simulink model "Adder"  (R2025a)
settings: Solver=FixedStepAuto  StartTime=0.0  StopTime=10.0  RelTol=1e-3
undefined symbols (not defined in the file or in its folder): A, B
libraries: hdlsllib x8
settings Model: Creator=Soochan Kim  LastModifiedBy=Soochan Kim
settings SolverCC: PositivePriorityOrder=on
settings OptimizationCC: BlockReduction=off  ConditionallyExecuteInputs=off  DefaultParameterBehavior=Inlined  EnhancedBackFolding=on  PassReuseOutputArgsAs=Individual arguments  ZeroExternalMemoryAtStartup=off  ZeroInternalMemoryAtStartup=off  MaxStackSize=64  OptimizeBlockOrder=speed  DifferentSizesBufferReuse=on  OptimizationCustomize=off  EfficientTunableParamExpr=on
settings DebuggingCC: AlgebraicLoopMsg=error  ParameterTunabilityLossMsg=error
settings HardwareCC: ProdBitPerPointer=32.0  ProdBitPerSizeT=32.0  ProdBitPerPtrDiffT=32.0  ProdLargestAtomicFloat=None  ProdIntDivRoundTo=Undefined  ProdEndianess=Unspecified  ProdWordSize=32.0  ProdHWDeviceType=ASIC/FPGA->ASIC/FPGA  TargetBitPerPointer=64.0  TargetBitPerSizeT=64.0  TargetBitPerPtrDiffT=64.0  TargetLongLongMode=on  TargetIntDivRoundTo=Zero  TargetEndianess=LittleEndian  TargetWordSize=64.0  TargetHWDeviceType=Custom Processor->MATLAB Host Computer  ProdEqTarget=off
settings SFSimCC: MATLABDynamicMemAlloc=off
settings RTWCC: SystemTargetFile=ert.tlc  TemplateMakefile=ert_default_tmf  Toolchain=ARM Development Studio Altera Edition (DS-5 AE)  Description=Embedded Coder
settings CodeAppCC: ForceParamTrailComments=on  IgnoreCustomStorageClasses=off  OperatorAnnotations=on  SimulinkDataObjDesc=on  SFDataObjDesc=on  InsertBlockDesc=on
settings ERTTargetCC: ExtModeTransport=0.0  ExtModeStaticAlloc=off  ExtModeMexFile=ext_comm  ExtModeIntrfLevel=Level1  ERTCustomFileTemplate=example_file_process.tlc

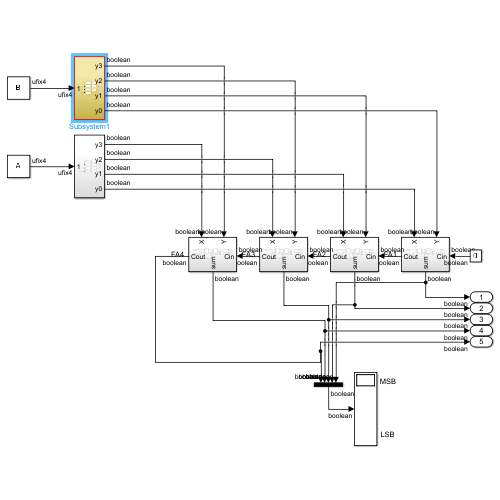
[thumbnail: Simulink's stored preview of the top-level diagram]
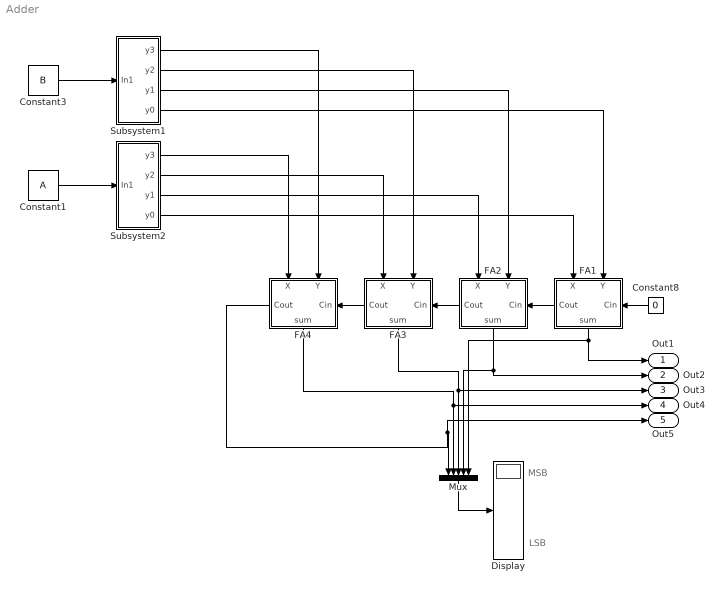
== system Adder ==
  note: MSB
  note: LSB
  Constant1 : Constant  Value=A  OutDataTypeStr=fixdt(0,4,0)  SampleTime=1
  Constant3 : Constant  Value=B  OutDataTypeStr=fixdt(0,4,0)  SampleTime=1
  Constant8 : Constant  Value=0  OutDataTypeStr=boolean  SampleTime=0
  Display : Display
  FA1 : Subsystem
      settings: PortSchema="{\"entries\":[{\"content\":{\"sides\":[{\"content\":{\"connectorIds\":[\"In1\",\"In2\"]},\"type\":\"ConnectorPlacement.EquallySpacedRectSide\",\"uuid\":\"42c5f982-256f-4156-9adc-36f89430248c\"},{\"content\":{\"connectorIds\":[\"Out1\"],\"side\":\"RIGHT\"},\"type\":\"ConnectorPlacement.EquallySpacedRectSide\",\"uuid\":\"9d11c24e-870a-4148-b8b5-25a7beca76ab\"},{\"content\":{\"connectorIds\":[\"Out2\"],\"side\":\"TOP\"},\"type\":\"ConnectorPlacement.EquallySpacedRectSide\",\"uuid\":\"c1f70d36-b796-4c24-b354-d6a39f97a60f\"},{\"content\":{\"connectorIds\":[\"In3\"],\"side\":\"BOTTOM\"},\"type\":\"ConnectorPlacement.EquallySpacedRectSide\",\"uuid\":\"4a8088db-d427-4c0f-97c8-d6eaf5b2c831\"}]},\"type\":\"ConnectorPlacement.EquallySpacedConnector\",\"uuid\":\"06197126-ee43-434f-a8ec-ad2442b26956\"}],\"packageUris\":[\"http://schema.mathworks.com/mf0/Connector/R2020b\"],\"version\":\"1.0\"}"
  FA2 : Subsystem
      settings: PortSchema="{\"entries\":[{\"content\":{\"sides\":[{\"content\":{\"connectorIds\":[\"In1\",\"In2\"]},\"type\":\"ConnectorPlacement.EquallySpacedRectSide\",\"uuid\":\"42c5f982-256f-4156-9adc-36f89430248c\"},{\"content\":{\"connectorIds\":[\"Out1\"],\"side\":\"RIGHT\"},\"type\":\"ConnectorPlacement.EquallySpacedRectSide\",\"uuid\":\"9d11c24e-870a-4148-b8b5-25a7beca76ab\"},{\"content\":{\"connectorIds\":[\"Out2\"],\"side\":\"TOP\"},\"type\":\"ConnectorPlacement.EquallySpacedRectSide\",\"uuid\":\"c1f70d36-b796-4c24-b354-d6a39f97a60f\"},{\"content\":{\"connectorIds\":[\"In3\"],\"side\":\"BOTTOM\"},\"type\":\"ConnectorPlacement.EquallySpacedRectSide\",\"uuid\":\"4a8088db-d427-4c0f-97c8-d6eaf5b2c831\"}]},\"type\":\"ConnectorPlacement.EquallySpacedConnector\",\"uuid\":\"06197126-ee43-434f-a8ec-ad2442b26956\"}],\"packageUris\":[\"http://schema.mathworks.com/mf0/Connector/R2020b\"],\"version\":\"1.0\"}"
  FA3 : Subsystem
      settings: PortSchema="{\"entries\":[{\"content\":{\"sides\":[{\"content\":{\"connectorIds\":[\"In1\",\"In2\"]},\"type\":\"ConnectorPlacement.EquallySpacedRectSide\",\"uuid\":\"42c5f982-256f-4156-9adc-36f89430248c\"},{\"content\":{\"connectorIds\":[\"Out1\"],\"side\":\"RIGHT\"},\"type\":\"ConnectorPlacement.EquallySpacedRectSide\",\"uuid\":\"9d11c24e-870a-4148-b8b5-25a7beca76ab\"},{\"content\":{\"connectorIds\":[\"Out2\"],\"side\":\"TOP\"},\"type\":\"ConnectorPlacement.EquallySpacedRectSide\",\"uuid\":\"c1f70d36-b796-4c24-b354-d6a39f97a60f\"},{\"content\":{\"connectorIds\":[\"In3\"],\"side\":\"BOTTOM\"},\"type\":\"ConnectorPlacement.EquallySpacedRectSide\",\"uuid\":\"4a8088db-d427-4c0f-97c8-d6eaf5b2c831\"}]},\"type\":\"ConnectorPlacement.EquallySpacedConnector\",\"uuid\":\"06197126-ee43-434f-a8ec-ad2442b26956\"}],\"packageUris\":[\"http://schema.mathworks.com/mf0/Connector/R2020b\"],\"version\":\"1.0\"}"
  FA4 : Subsystem
      settings: PortSchema="{\"entries\":[{\"content\":{\"sides\":[{\"content\":{\"connectorIds\":[\"In1\",\"In2\"]},\"type\":\"ConnectorPlacement.EquallySpacedRectSide\",\"uuid\":\"42c5f982-256f-4156-9adc-36f89430248c\"},{\"content\":{\"connectorIds\":[\"Out1\"],\"side\":\"RIGHT\"},\"type\":\"ConnectorPlacement.EquallySpacedRectSide\",\"uuid\":\"9d11c24e-870a-4148-b8b5-25a7beca76ab\"},{\"content\":{\"connectorIds\":[\"Out2\"],\"side\":\"TOP\"},\"type\":\"ConnectorPlacement.EquallySpacedRectSide\",\"uuid\":\"c1f70d36-b796-4c24-b354-d6a39f97a60f\"},{\"content\":{\"connectorIds\":[\"In3\"],\"side\":\"BOTTOM\"},\"type\":\"ConnectorPlacement.EquallySpacedRectSide\",\"uuid\":\"4a8088db-d427-4c0f-97c8-d6eaf5b2c831\"}]},\"type\":\"ConnectorPlacement.EquallySpacedConnector\",\"uuid\":\"06197126-ee43-434f-a8ec-ad2442b26956\"}],\"packageUris\":[\"http://schema.mathworks.com/mf0/Connector/R2020b\"],\"version\":\"1.0\"}"
  Mux : Mux  Inputs=5
  Subsystem1 : Subsystem
  Subsystem2 : Subsystem
  Out1 : Outport  VectorParamsAs1DForOutWhenUnconnected=off
  Out2 : Outport  Port=2  VectorParamsAs1DForOutWhenUnconnected=off
  Out3 : Outport  Port=3  VectorParamsAs1DForOutWhenUnconnected=off
  Out4 : Outport  Port=4  VectorParamsAs1DForOutWhenUnconnected=off
  Out5 : Outport  Port=5  VectorParamsAs1DForOutWhenUnconnected=off
  wires:
  FA1/2(Cout) -> FA2/3(Cin)
  FA2/2(Cout) -> FA3/3(Cin)
  FA3/2(Cout) -> FA4/3(Cin)
  FA1/1(sum) -> Out1/1, Mux/5
  FA2/1(sum) -> Out2/1, Mux/4
  FA3/1(sum) -> Out3/1, Mux/3
  FA4/1(sum) -> Out4/1, Mux/2
  FA4/2(Cout) -> Out5/1, Mux/1
  Constant8/1 -> FA1/3(Cin)
  Subsystem2/1(y3) -> FA4/1(X)
  Subsystem2/2(y2) -> FA3/1(X)
  Subsystem2/3(y1) -> FA2/1(X)
  Subsystem2/4(y0) -> FA1/1(X)
  Subsystem1/1(y3) -> FA4/2(Y)
  Subsystem1/2(y2) -> FA3/2(Y)
  Subsystem1/3(y1) -> FA2/2(Y)
  Subsystem1/4(y0) -> FA1/2(Y)
  Mux/1 -> Display/1
  Constant1/1 -> Subsystem2/1(In1)
  Constant3/1 -> Subsystem1/1(In1)

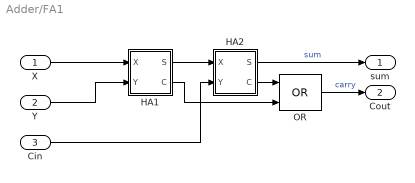
== system Adder/FA1 ==
  X : Inport
  Y : Inport  Port=2
  Cin : Inport  Port=3
  HA1 : Subsystem
  HA2 : Subsystem
  OR : Logic  Operator=OR  IconShape=distinctive  AllPortsSameDT=off  OutDataTypeStr=boolean
  sum : Outport
  Cout : Outport  Port=2
  wires:
  HA2/2(C) -> OR/1
  X/1 -> HA1/1(X)
  HA1/2(C) -> OR/2
  Y/1 -> HA1/2(Y)
  Cin/1 -> HA2/2(Y)
  HA1/1(S) -> HA2/1(X)
  OR/1 -> Cout/1  "carry"
  HA2/1(S) -> sum/1  "sum"

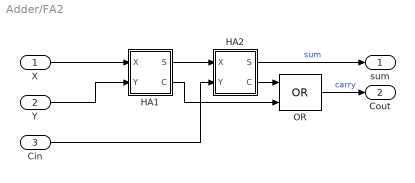
== system Adder/FA2 ==
  X : Inport
  Y : Inport  Port=2
  Cin : Inport  Port=3
  HA1 : Subsystem
  HA2 : Subsystem
  OR : Logic  Operator=OR  IconShape=distinctive  AllPortsSameDT=off  OutDataTypeStr=boolean
  sum : Outport
  Cout : Outport  Port=2
  wires:
  HA2/2(C) -> OR/1
  X/1 -> HA1/1(X)
  HA1/2(C) -> OR/2
  Y/1 -> HA1/2(Y)
  Cin/1 -> HA2/2(Y)
  HA1/1(S) -> HA2/1(X)
  OR/1 -> Cout/1  "carry"
  HA2/1(S) -> sum/1  "sum"

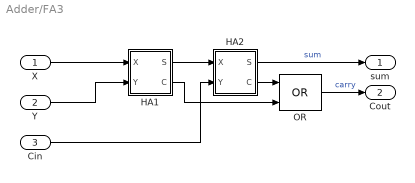
== system Adder/FA3 ==
  X : Inport
  Y : Inport  Port=2
  Cin : Inport  Port=3
  HA1 : Subsystem
  HA2 : Subsystem
  OR : Logic  Operator=OR  IconShape=distinctive  AllPortsSameDT=off  OutDataTypeStr=boolean
  sum : Outport
  Cout : Outport  Port=2
  wires:
  HA2/2(C) -> OR/1
  X/1 -> HA1/1(X)
  HA1/2(C) -> OR/2
  Y/1 -> HA1/2(Y)
  Cin/1 -> HA2/2(Y)
  HA1/1(S) -> HA2/1(X)
  OR/1 -> Cout/1  "carry"
  HA2/1(S) -> sum/1  "sum"

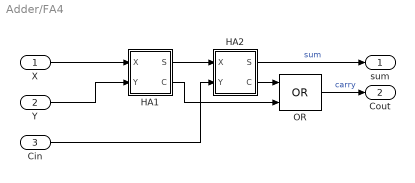
== system Adder/FA4 ==
  X : Inport
  Y : Inport  Port=2
  Cin : Inport  Port=3
  HA1 : Subsystem
  HA2 : Subsystem
  OR : Logic  Operator=OR  IconShape=distinctive  AllPortsSameDT=off  OutDataTypeStr=boolean
  sum : Outport
  Cout : Outport  Port=2
  wires:
  HA2/2(C) -> OR/1
  X/1 -> HA1/1(X)
  HA1/2(C) -> OR/2
  Y/1 -> HA1/2(Y)
  Cin/1 -> HA2/2(Y)
  HA1/1(S) -> HA2/1(X)
  OR/1 -> Cout/1  "carry"
  HA2/1(S) -> sum/1  "sum"

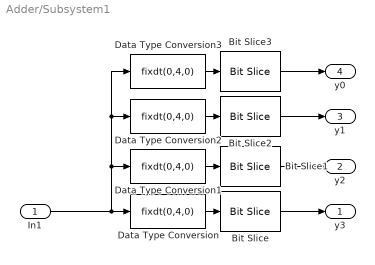
== system Adder/Subsystem1 ==
  In1 : Inport
  Bit Slice : hdlsllib/Logic and Bit Operations/Bit Slice  lidx=3  ridx=3
  Bit Slice1 : hdlsllib/Logic and Bit Operations/Bit Slice  lidx=2  ridx=2
  Bit Slice2 : hdlsllib/Logic and Bit Operations/Bit Slice  lidx=1  ridx=1
  Bit Slice3 : hdlsllib/Logic and Bit Operations/Bit Slice  lidx=0  ridx=0
  Data Type Conversion{,1..3} (4 alike) : DataTypeConversion  OutDataTypeStr=fixdt(0,4,0)  ConvertRealWorld=Stored Integer (SI)  RndMeth=Floor
  y3 : Outport  OutDataTypeStr=boolean
  y2 : Outport  Port=2  OutDataTypeStr=boolean
  y1 : Outport  Port=3  OutDataTypeStr=boolean
  y0 : Outport  Port=4  OutDataTypeStr=boolean
  wires:
  Bit Slice3/1 -> y0/1
  Bit Slice/1 -> y3/1
  Bit Slice1/1 -> y2/1
  Data Type Conversion3/1 -> Bit Slice3/1
  Data Type Conversion2/1 -> Bit Slice2/1
  Data Type Conversion/1 -> Bit Slice/1
  In1/1 -> Data Type Conversion/1, Data Type Conversion1/1, Data Type Conversion3/1, Data Type Conversion2/1
  Data Type Conversion1/1 -> Bit Slice1/1
  Bit Slice2/1 -> y1/1

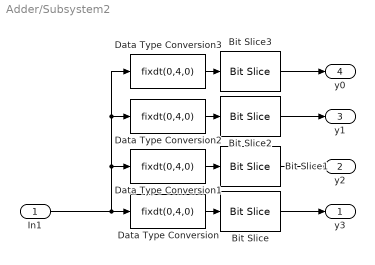
== system Adder/Subsystem2 ==
  In1 : Inport
  Bit Slice : hdlsllib/Logic and Bit Operations/Bit Slice  lidx=3  ridx=3
  Bit Slice1 : hdlsllib/Logic and Bit Operations/Bit Slice  lidx=2  ridx=2
  Bit Slice2 : hdlsllib/Logic and Bit Operations/Bit Slice  lidx=1  ridx=1
  Bit Slice3 : hdlsllib/Logic and Bit Operations/Bit Slice  lidx=0  ridx=0
  Data Type Conversion{,1..3} (4 alike) : DataTypeConversion  OutDataTypeStr=fixdt(0,4,0)  ConvertRealWorld=Stored Integer (SI)  RndMeth=Floor
  y3 : Outport  OutDataTypeStr=boolean
  y2 : Outport  Port=2  OutDataTypeStr=boolean
  y1 : Outport  Port=3  OutDataTypeStr=boolean
  y0 : Outport  Port=4  OutDataTypeStr=boolean
  wires:
  Bit Slice3/1 -> y0/1
  Bit Slice/1 -> y3/1
  Bit Slice1/1 -> y2/1
  Data Type Conversion3/1 -> Bit Slice3/1
  Data Type Conversion2/1 -> Bit Slice2/1
  Data Type Conversion/1 -> Bit Slice/1
  In1/1 -> Data Type Conversion/1, Data Type Conversion1/1, Data Type Conversion3/1, Data Type Conversion2/1
  Data Type Conversion1/1 -> Bit Slice1/1
  Bit Slice2/1 -> y1/1

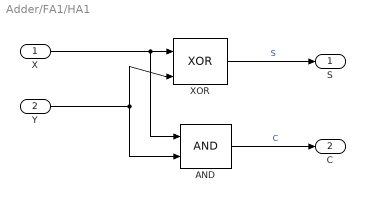
== system Adder/FA1/HA1 ==
  X : Inport
  Y : Inport  Port=2
  AND : Logic  IconShape=distinctive  AllPortsSameDT=off  OutDataTypeStr=boolean
  XOR : Logic  Operator=XOR  IconShape=distinctive  AllPortsSameDT=off  OutDataTypeStr=boolean
  S : Outport
  C : Outport  Port=2
  wires:
  Y/1 -> XOR/2, AND/2
  XOR/1 -> S/1  "S"
  X/1 -> AND/1, XOR/1
  AND/1 -> C/1  "C"

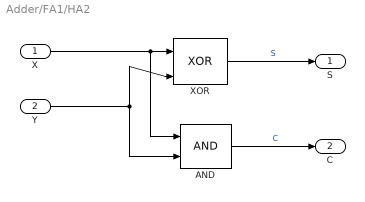
== system Adder/FA1/HA2 ==
  X : Inport
  Y : Inport  Port=2
  AND : Logic  IconShape=distinctive  AllPortsSameDT=off  OutDataTypeStr=boolean
  XOR : Logic  Operator=XOR  IconShape=distinctive  AllPortsSameDT=off  OutDataTypeStr=boolean
  S : Outport
  C : Outport  Port=2
  wires:
  Y/1 -> XOR/2, AND/2
  XOR/1 -> S/1  "S"
  X/1 -> AND/1, XOR/1
  AND/1 -> C/1  "C"

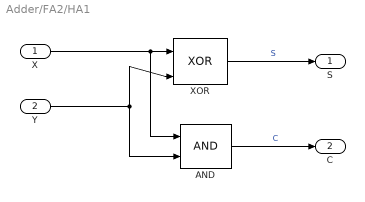
== system Adder/FA2/HA1 ==
  X : Inport
  Y : Inport  Port=2
  AND : Logic  IconShape=distinctive  AllPortsSameDT=off  OutDataTypeStr=boolean
  XOR : Logic  Operator=XOR  IconShape=distinctive  AllPortsSameDT=off  OutDataTypeStr=boolean
  S : Outport
  C : Outport  Port=2
  wires:
  Y/1 -> XOR/2, AND/2
  XOR/1 -> S/1  "S"
  X/1 -> AND/1, XOR/1
  AND/1 -> C/1  "C"

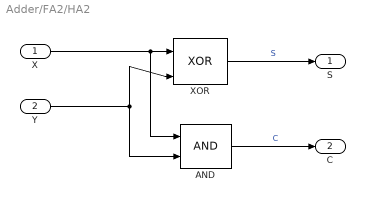
== system Adder/FA2/HA2 ==
  X : Inport
  Y : Inport  Port=2
  AND : Logic  IconShape=distinctive  AllPortsSameDT=off  OutDataTypeStr=boolean
  XOR : Logic  Operator=XOR  IconShape=distinctive  AllPortsSameDT=off  OutDataTypeStr=boolean
  S : Outport
  C : Outport  Port=2
  wires:
  Y/1 -> XOR/2, AND/2
  XOR/1 -> S/1  "S"
  X/1 -> AND/1, XOR/1
  AND/1 -> C/1  "C"

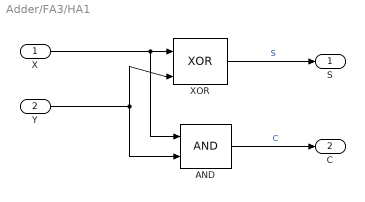
== system Adder/FA3/HA1 ==
  X : Inport
  Y : Inport  Port=2
  AND : Logic  IconShape=distinctive  AllPortsSameDT=off  OutDataTypeStr=boolean
  XOR : Logic  Operator=XOR  IconShape=distinctive  AllPortsSameDT=off  OutDataTypeStr=boolean
  S : Outport
  C : Outport  Port=2
  wires:
  Y/1 -> XOR/2, AND/2
  XOR/1 -> S/1  "S"
  X/1 -> AND/1, XOR/1
  AND/1 -> C/1  "C"

== system Adder/FA3/HA2 ==
  X : Inport
  Y : Inport  Port=2
  AND : Logic  IconShape=distinctive  AllPortsSameDT=off  OutDataTypeStr=boolean
  XOR : Logic  Operator=XOR  IconShape=distinctive  AllPortsSameDT=off  OutDataTypeStr=boolean
  S : Outport
  C : Outport  Port=2
  wires:
  Y/1 -> XOR/2, AND/2
  XOR/1 -> S/1  "S"
  X/1 -> AND/1, XOR/1
  AND/1 -> C/1  "C"

== system Adder/FA4/HA1 ==
  X : Inport
  Y : Inport  Port=2
  AND : Logic  IconShape=distinctive  AllPortsSameDT=off  OutDataTypeStr=boolean
  XOR : Logic  Operator=XOR  IconShape=distinctive  AllPortsSameDT=off  OutDataTypeStr=boolean
  S : Outport
  C : Outport  Port=2
  wires:
  Y/1 -> XOR/2, AND/2
  XOR/1 -> S/1  "S"
  X/1 -> AND/1, XOR/1
  AND/1 -> C/1  "C"

== system Adder/FA4/HA2 ==
  X : Inport
  Y : Inport  Port=2
  AND : Logic  IconShape=distinctive  AllPortsSameDT=off  OutDataTypeStr=boolean
  XOR : Logic  Operator=XOR  IconShape=distinctive  AllPortsSameDT=off  OutDataTypeStr=boolean
  S : Outport
  C : Outport  Port=2
  wires:
  Y/1 -> XOR/2, AND/2
  XOR/1 -> S/1  "S"
  X/1 -> AND/1, XOR/1
  AND/1 -> C/1  "C"
